simulink model "ac_generator_feedback_R2018a"  (R2018a)
settings: Solver=ode15s  StartTime=0.0  StopTime=12  MaxStep=1e-3  RelTol=1e-3
undefined symbols (not defined in the file or in its folder): C, D, f_gen, Gamma, h, J_gen, K_gen, Kv, l0, Lv, n, Phi, w_g
settings Model: Creator=kjartan  LastModifiedBy=kjartan
settings DataIOCC: ReturnWorkspaceOutputs=on
settings DebuggingCC: UnconnectedInputMsg=none  UnconnectedOutputMsg=none  UnconnectedLineMsg=none  SFMachineParentedDataDiag=error
settings ModelReferenceCC: EnableRefExpFcnMdlSchedulingChecks=off
settings SFSimCC: SimUseLocalCustomCode=on
settings RTWCC: Description=Generic Real-Time Target  RTWUseLocalCustomCode=on

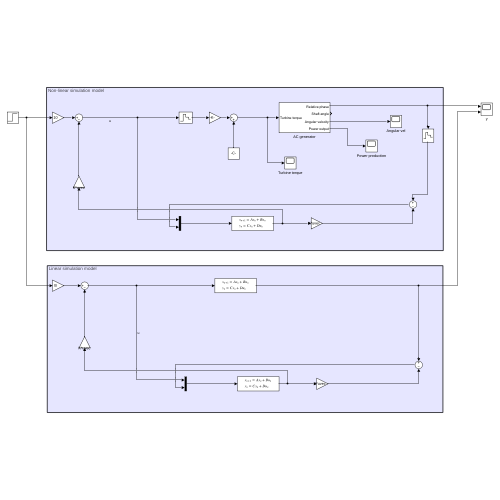
[thumbnail: Simulink's stored preview of the top-level diagram]
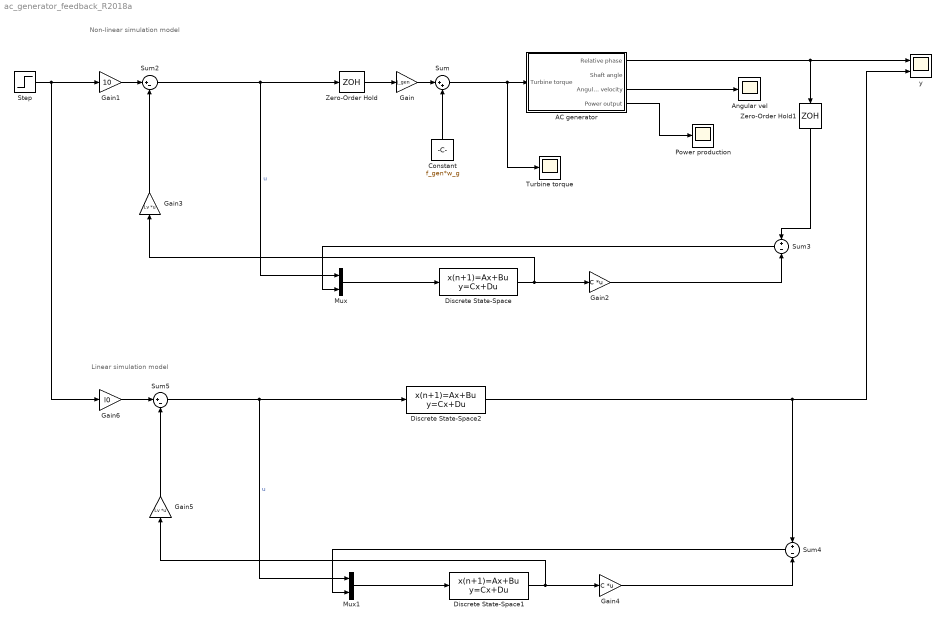
== system ac_generator_feedback_R2018a ==
  note: Linear simulation model
  note: Non-linear simulation model
  AC generator : Subsystem
  Angular vel : Scope
  Constant : Constant  Value=f_gen*w_g
  Discrete State-Space : DiscreteStateSpace  A=Phi  B=[Gamma, Kv]  C=eye(n)  D=zeros(n, 2)  SampleTime=h
  Discrete State-Space1 : DiscreteStateSpace  A=Phi  B=[Gamma, Kv]  C=eye(n)  D=zeros(n, 2)  SampleTime=h
  Discrete State-Space2 : DiscreteStateSpace  A=Phi  B=Gamma  C=C  D=D  SampleTime=h
  Gain : Gain  Gain=J_gen
  Gain1 : Gain  Gain=10
  Gain2 : Gain  Gain=C  Multiplication=Matrix(K*u) (u vector)
  Gain3 : Gain  Gain=Lv  Multiplication=Matrix(K*u) (u vector)
  Gain4 : Gain  Gain=C  Multiplication=Matrix(K*u) (u vector)
  Gain5 : Gain  Gain=Lv  Multiplication=Matrix(K*u) (u vector)
  Gain6 : Gain  Gain=l0
  Mux : Mux  Inputs=2
  Mux1 : Mux  Inputs=2
  Power production : Scope
  Step : Step  After=0.3  SampleTime=0
  Sum : Sum  Inputs=|++
  Sum2 : Sum  Inputs=|+-
  Sum3 : Sum  Inputs=+|-
  Sum4 : Sum  Inputs=+|-
  Sum5 : Sum  Inputs=|+-
  Turbine torque : Scope
  Zero-Order Hold : ZeroOrderHold  SampleTime=h
  Zero-Order Hold1 : ZeroOrderHold  SampleTime=h
  y : Scope  NumInputPorts=2
  wires:
  AC generator/1(Relative phase) -> y/1, Zero-Order Hold1/1
  Sum2/1 -> Zero-Order Hold/1, Mux/1  "u"
  AC generator/3(Angular velocity) -> Angular vel/1
  AC generator/4(Power output) -> Power production/1
  Constant/1 -> Sum/2
  Gain/1 -> Sum/1
  Zero-Order Hold/1 -> Gain/1
  Step/1 -> Gain6/1, Gain1/1
  Gain1/1 -> Sum2/1
  Discrete State-Space/1 -> Gain2/1, Gain3/1
  Gain2/1 -> Sum3/2
  Sum3/1 -> Mux/2
  Mux/1 -> Discrete State-Space/1
  Gain3/1 -> Sum2/2
  Zero-Order Hold1/1 -> Sum3/1
  Mux1/1 -> Discrete State-Space1/1
  Sum4/1 -> Mux1/2
  Discrete State-Space1/1 -> Gain4/1, Gain5/1
  Gain5/1 -> Sum5/2
  Sum5/1 -> Discrete State-Space2/1, Mux1/1  "u"
  Gain4/1 -> Sum4/2
  Discrete State-Space2/1 -> y/2, Sum4/1
  Gain6/1 -> Sum5/1
  Sum/1 -> Turbine torque/1, AC generator/1(Turbine torque)

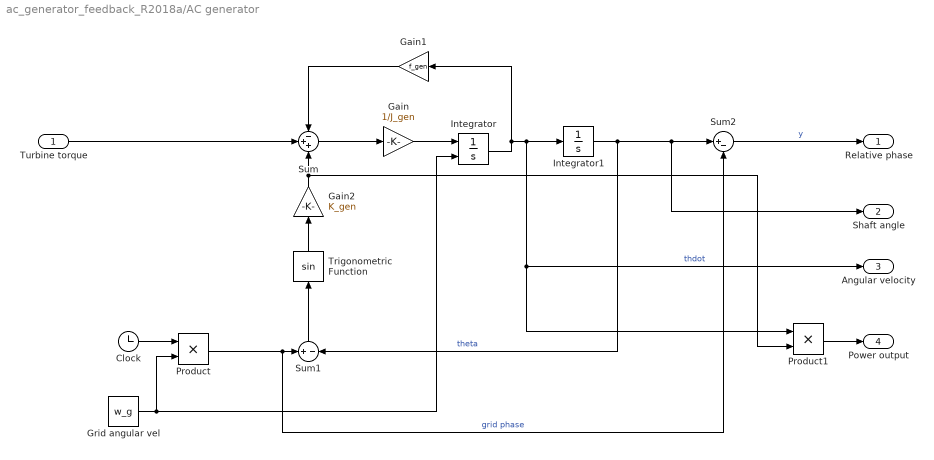
== system ac_generator_feedback_R2018a/AC generator ==
  Turbine torque : Inport
  Clock : Clock
  Gain : Gain  Gain=1/J_gen
  Gain1 : Gain  Gain=f_gen
  Gain2 : Gain  Gain=K_gen
  Grid angular vel : Constant  Value=w_g
  Integrator : Integrator  InitialConditionSource=external
  Integrator1 : Integrator
  Product : Product
  Product1 : Product
  Sum : Sum  Inputs=-++
  Sum1 : Sum  Inputs=+|-
  Sum2 : Sum  Inputs=|+-
  Trigonometric Function : Trigonometry
  Relative phase : Outport
  Shaft angle : Outport  Port=2
  Angular velocity : Outport  Port=3
  Power output : Outport  Port=4
  wires:
  Integrator1/1 -> Shaft angle/1, Sum2/1, Sum1/2  "theta"
  Sum2/1 -> Relative phase/1  "y"
  Gain1/1 -> Sum/1
  Gain2/1 -> Sum/3, Product1/2
  Product/1 -> Sum2/2, Sum1/1  "grid phase"
  Gain/1 -> Integrator/1
  Turbine torque/1 -> Sum/2
  Sum/1 -> Gain/1
  Clock/1 -> Product/1
  Integrator/1 -> Gain1/1, Product1/1, Angular velocity/1, Integrator1/1  "thdot"
  Grid angular vel/1 -> Integrator/2, Product/2
  Product1/1 -> Power output/1
  Sum1/1 -> Trigonometric Function/1
  Trigonometric Function/1 -> Gain2/1
